simulink library "lib_gyro_fusion"  (R2014a)
settings: Solver=ode45  StartTime=0.0  StopTime=10.0  RelTol=1e-3
undefined symbols (not defined in the file): acc_I, omega_B_noise, omega_bias_I_noise, q_noise, R_gyro
libraries: lib_gyro_fusion x16, aerolibnav x1, simulink x1, vrlib x1
settings Model: Creator=kirill  LastModifiedBy=kirill

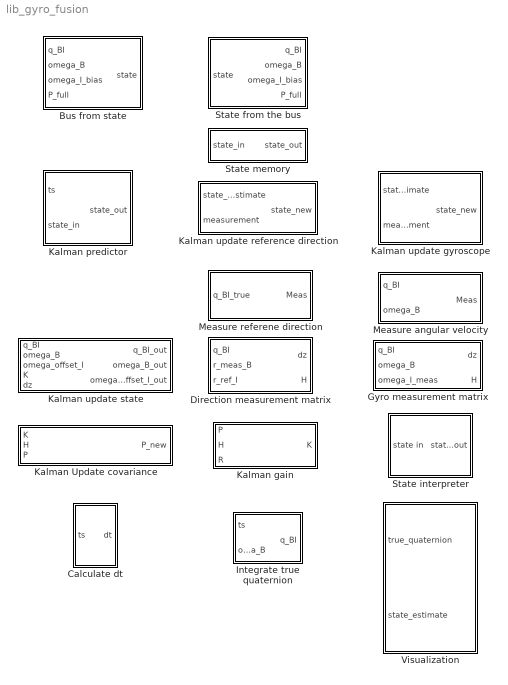
== system lib_gyro_fusion ==
  Bus from state : Subsystem
  Calculate dt : Subsystem
  Direction measurement matrix : Subsystem
  Gyro measurement matrix : Subsystem
  Integrate true quaternion : Subsystem  mask{q_BI_init=[1; 0; 0; 0]}
      mask prompts: q_BI_init "Initial quaternion"
  Kalman Update covariance : MATLAB Function  TreatAsAtomicUnit=on
  Kalman gain : MATLAB Function  TreatAsAtomicUnit=on
  Kalman predictor : Subsystem  mask{q_noise=q_noise, omega_B_noise=omega_B_noise, omega_I_bias_noise=omega_bias_I_noise}
      mask prompts: q_noise "Quaternion dynamics noise [rad/s]"; omega_B_noise "Angular velocity noise [x, y, z], [rad/s^2]"; omega_I_bias_noise "Angular velocity offset noise [rad/s^2]"
  Kalman update gyroscope : Subsystem
  Kalman update reference direction : Subsystem
  Kalman update state : Subsystem
  Measure angular velocity : Subsystem
  Measure referene direction : Subsystem  mask{ref_direction=[1; 0; 0], measurement_noise_power=[1, 1, 1] * 1e-4, measurement_sample_rate=0.1, source_seeds=[340901, 234090, 334090], R_direction=eye(3)}
      mask prompts: ref_direction "Reference direction (inertial frame)"; measurement_noise_power "Measurement noise power"; measurement_sample_rate "Measurement sample rate (seconds)"; source_seeds "Measurement random seeds"; R_direction "Direction measurement covariance covariance"
  State from the bus : Subsystem
  State interpreter : Subsystem
  State memory : Subsystem  mask{q_BI_init=[1; 0; 0; 0], omega_B_init=[0; 0; 0], omega_I_bias_init=[0; 0; 0], P_full_init=eye(9)}
      mask prompts: q_BI_init "Initial quaternion q_BI (4-column vector)"; omega_B_init "Initial body frame angular velocity"; omega_I_bias_init "Initial gyroscope bias (inertial reference frame)"; P_full_init "Initial full state covariance (9x9)"
  Visualization : Subsystem

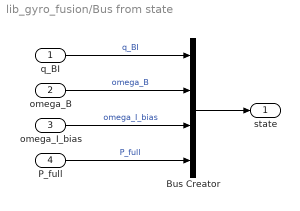
== system lib_gyro_fusion/Bus from state ==
  q_BI : Inport
  omega_B : Inport  Port=2
  omega_I_bias : Inport  Port=3
  P_full : Inport  Port=4
  Bus Creator : BusCreator
  state : Outport
  wires:
  omega_I_bias/1 -> Bus Creator/3  "omega_I_bias"
  P_full/1 -> Bus Creator/4  "P_full"
  q_BI/1 -> Bus Creator/1  "q_BI"
  omega_B/1 -> Bus Creator/2  "omega_B"
  Bus Creator/1 -> state/1

== system lib_gyro_fusion/Calculate dt ==
  ts : Inport
  Calculate dt : Sum  Inputs=+-
  Unit Delay : UnitDelay  SampleTime=-1
  dt : Outport
  wires:
  Unit Delay/1 -> Calculate dt/2
  Calculate dt/1 -> dt/1
  ts/1 -> Calculate dt/1, Unit Delay/1

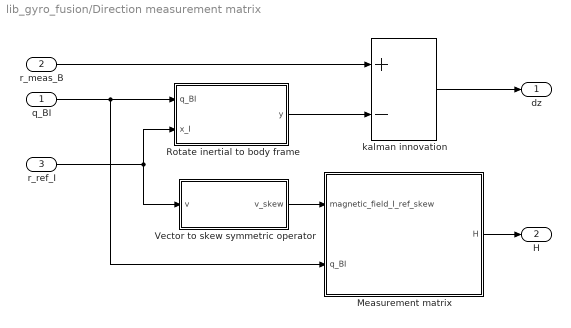
== system lib_gyro_fusion/Direction measurement matrix ==
  q_BI : Inport
  r_meas_B : Inport  Port=2
  r_ref_I : Inport  Port=3
  Measurement matrix : MATLAB Function  TreatAsAtomicUnit=on
  Rotate inertial to body frame : MATLAB Function  TreatAsAtomicUnit=on
  Vector to skew symmetric operator : MATLAB Function  TreatAsAtomicUnit=on
  kalman innovation : Sum  Inputs=+-
  dz : Outport
  H : Outport  Port=2
  wires:
  q_BI/1 -> Measurement matrix/2(q_BI), Rotate inertial to body frame/1(q_BI)
  r_ref_I/1 -> Rotate inertial to body frame/2(x_I), Vector to skew symmetric operator/1(v)
  Rotate inertial to body frame/1(y) -> kalman innovation/2
  r_meas_B/1 -> kalman innovation/1
  kalman innovation/1 -> dz/1
  Vector to skew symmetric operator/1(v_skew) -> Measurement matrix/1(magnetic_field_I_ref_skew)
  Measurement matrix/1(H) -> H/1

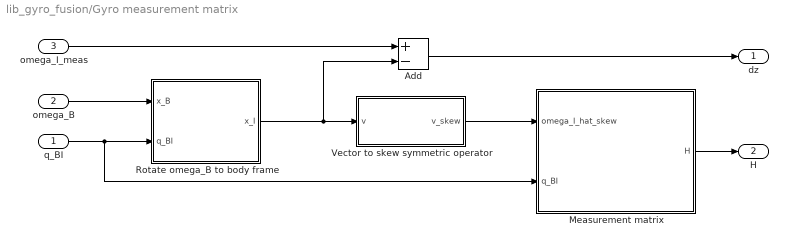
== system lib_gyro_fusion/Gyro measurement matrix ==
  q_BI : Inport
  omega_B : Inport  Port=2
  omega_I_meas : Inport  Port=3
  Add : Sum  Inputs=+-
  Measurement matrix : MATLAB Function  TreatAsAtomicUnit=on
  Rotate omega_B to body frame : MATLAB Function  TreatAsAtomicUnit=on
  Vector to skew symmetric operator : MATLAB Function  TreatAsAtomicUnit=on
  dz : Outport
  H : Outport  Port=2
  wires:
  Add/1 -> dz/1
  omega_I_meas/1 -> Add/1
  q_BI/1 -> Rotate omega_B to body frame/2(q_BI), Measurement matrix/2(q_BI)
  Vector to skew symmetric operator/1(v_skew) -> Measurement matrix/1(omega_I_hat_skew)
  Measurement matrix/1(H) -> H/1
  Rotate omega_B to body frame/1(x_I) -> Add/2, Vector to skew symmetric operator/1(v)
  omega_B/1 -> Rotate omega_B to body frame/1(x_B)

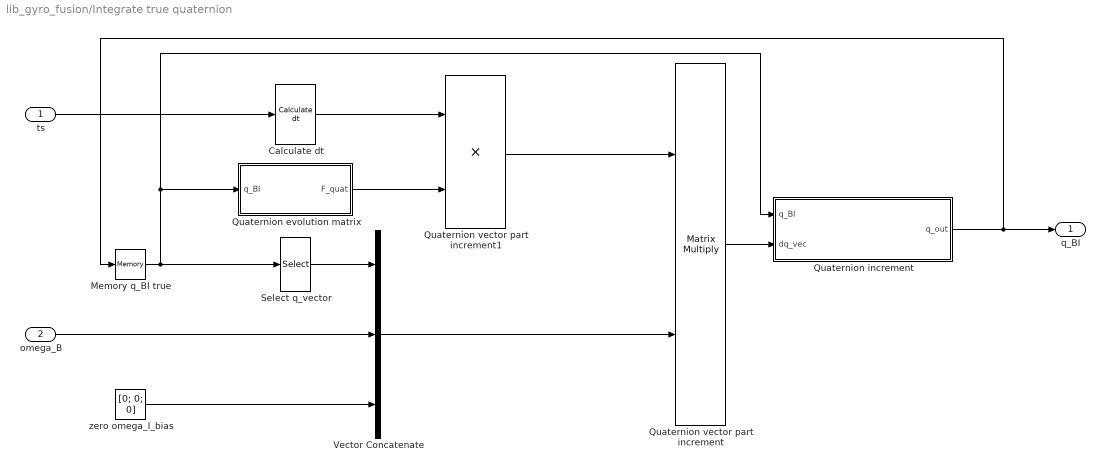
== system lib_gyro_fusion/Integrate true quaternion ==
  ts : Inport
  omega_B : Inport  Port=2
  Calculate dt : lib_gyro_fusion/Calculate dt
  Memory q_BI true : Memory  X0=q_BI_init
  Quaternion evolution matrix : MATLAB Function  TreatAsAtomicUnit=on
  Quaternion increment : MATLAB Function  TreatAsAtomicUnit=on
  Quaternion vector part increment : Product  Multiplication=Matrix(*)
  Quaternion vector part increment1 : Product
  Select q_vector : Selector  InputPortWidth=4  IndexOptions=Starting index (dialog)  Indices=2  OutputSizes=3
  Vector Concatenate : Concatenate  NumInputs=3
  zero omega_I_bias : Constant  Value=[0; 0; 0]
  q_BI : Outport
  wires:
  Quaternion vector part increment/1 -> Quaternion increment/2(dq_vec)
  zero omega_I_bias/1 -> Vector Concatenate/3
  Vector Concatenate/1 -> Quaternion vector part increment/2
  omega_B/1 -> Vector Concatenate/2
  Quaternion evolution matrix/1(F_quat) -> Quaternion vector part increment1/2
  Calculate dt/1 -> Quaternion vector part increment1/1
  Quaternion increment/1(q_out) -> q_BI/1, Memory q_BI true/1
  Memory q_BI true/1 -> Quaternion increment/1(q_BI), Quaternion evolution matrix/1(q_BI), Select q_vector/1
  Quaternion vector part increment1/1 -> Quaternion vector part increment/1
  ts/1 -> Calculate dt/1
  Select q_vector/1 -> Vector Concatenate/1

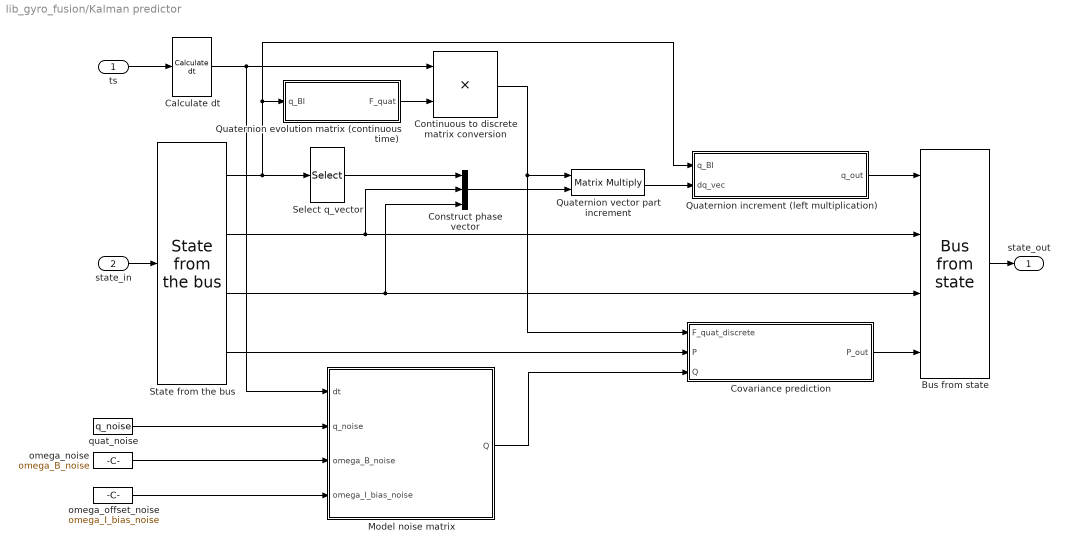
== system lib_gyro_fusion/Kalman predictor ==
  ts : Inport
  state_in : Inport  Port=2
  Bus from state : lib_gyro_fusion/Bus from state
  Calculate dt : lib_gyro_fusion/Calculate dt
  Construct phase vector : Concatenate  NumInputs=3
  Continuous to discrete matrix conversion : Product
  Covariance prediction : MATLAB Function  TreatAsAtomicUnit=on
  Model noise matrix : MATLAB Function  TreatAsAtomicUnit=on
  Quaternion evolution matrix (continuous time) : MATLAB Function  TreatAsAtomicUnit=on
  Quaternion increment (left multiplication) : MATLAB Function  TreatAsAtomicUnit=on
  Quaternion vector part increment : Product  Multiplication=Matrix(*)
  Select q_vector : Selector  InputPortWidth=4  IndexOptions=Starting index (dialog)  Indices=2  OutputSizes=3
  State from the bus : lib_gyro_fusion/State from the bus
  omega_noise : Constant  Value=omega_B_noise
  omega_offset_noise : Constant  Value=omega_I_bias_noise
  quat_noise : Constant  Value=q_noise
  state_out : Outport
  wires:
  omega_offset_noise/1 -> Model noise matrix/4(omega_I_bias_noise)
  omega_noise/1 -> Model noise matrix/3(omega_B_noise)
  Calculate dt/1 -> Continuous to discrete matrix conversion/1, Model noise matrix/1(dt)
  quat_noise/1 -> Model noise matrix/2(q_noise)
  Model noise matrix/1(Q) -> Covariance prediction/3(Q)
  Covariance prediction/1(P_out) -> Bus from state/4
  State from the bus/4 -> Covariance prediction/2(P)
  Construct phase vector/1 -> Quaternion vector part increment/2
  Continuous to discrete matrix conversion/1 -> Quaternion vector part increment/1, Covariance prediction/1(F_quat_discrete)
  Quaternion evolution matrix (continuous time)/1(F_quat) -> Continuous to discrete matrix conversion/2
  Quaternion vector part increment/1 -> Quaternion increment (left multiplication)/2(dq_vec)
  Select q_vector/1 -> Construct phase vector/1
  State from the bus/1 -> Select q_vector/1, Quaternion evolution matrix (continuous time)/1(q_BI), Quaternion increment (left multiplication)/1(q_BI)
  ts/1 -> Calculate dt/1
  Quaternion increment (left multiplication)/1(q_out) -> Bus from state/1
  State from the bus/2 -> Construct phase vector/2, Bus from state/2
  State from the bus/3 -> Bus from state/3, Construct phase vector/3
  Bus from state/1 -> state_out/1
  state_in/1 -> State from the bus/1

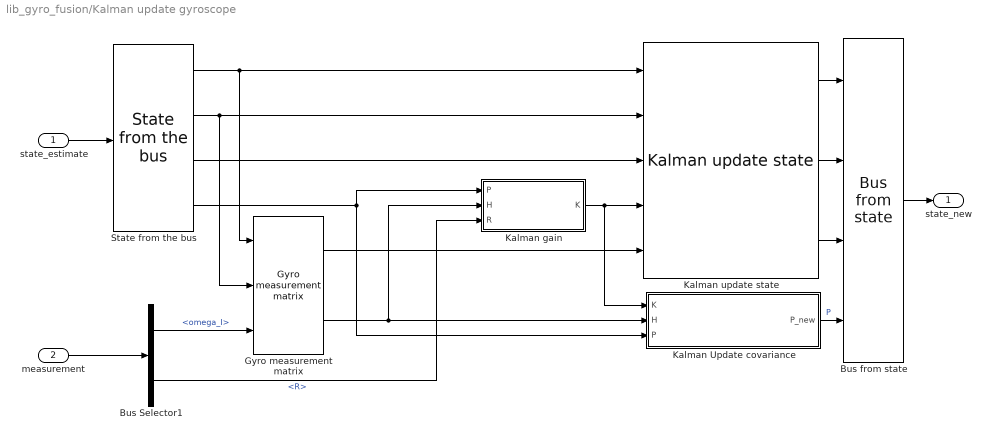
== system lib_gyro_fusion/Kalman update gyroscope ==
  state_estimate : Inport
  measurement : Inport  Port=2
  Bus Selector1 : BusSelector  OutputSignals=omega_I,R
  Bus from state : lib_gyro_fusion/Bus from state
  Gyro measurement matrix : lib_gyro_fusion/Gyro measurement matrix
  Kalman Update covariance : MATLAB Function  TreatAsAtomicUnit=on
  Kalman gain : MATLAB Function  TreatAsAtomicUnit=on
  Kalman update state : lib_gyro_fusion/Kalman update state
  State from the bus : lib_gyro_fusion/State from the bus
  state_new : Outport
  wires:
  Kalman update state/2 -> Bus from state/2
  Bus Selector1/2 -> Kalman gain/3(R)  "<R>"
  Kalman update state/3 -> Bus from state/3
  Kalman update state/1 -> Bus from state/1
  Gyro measurement matrix/1 -> Kalman update state/5
  Kalman gain/1(K) -> Kalman update state/4, Kalman Update covariance/1(K)
  State from the bus/3 -> Kalman update state/3
  State from the bus/2 -> Gyro measurement matrix/2, Kalman update state/2
  Gyro measurement matrix/2 -> Kalman gain/2(H), Kalman Update covariance/2(H)
  Bus Selector1/1 -> Gyro measurement matrix/3  "<omega_I>"
  State from the bus/1 -> Gyro measurement matrix/1, Kalman update state/1
  State from the bus/4 -> Kalman gain/1(P), Kalman Update covariance/3(P)
  state_estimate/1 -> State from the bus/1
  measurement/1 -> Bus Selector1/1
  Kalman Update covariance/1(P_new) -> Bus from state/4  "P"
  Bus from state/1 -> state_new/1

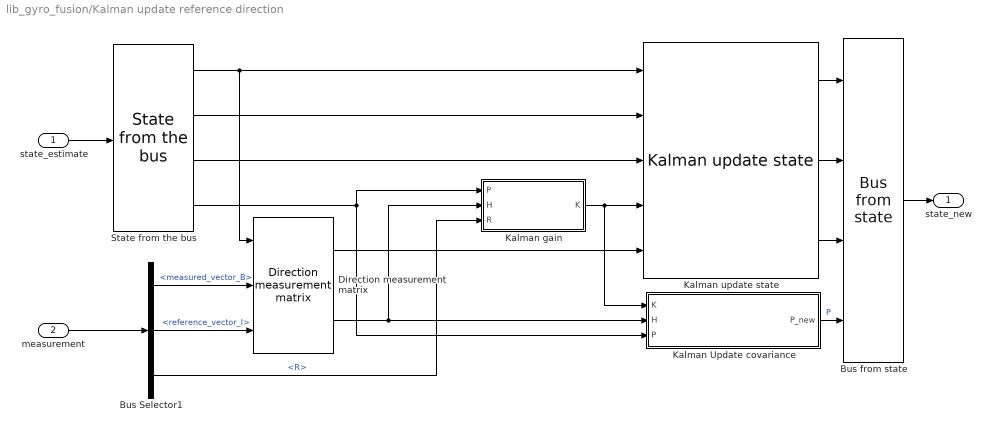
== system lib_gyro_fusion/Kalman update reference direction ==
  state_estimate : Inport
  measurement : Inport  Port=2
  Bus Selector1 : BusSelector  OutputSignals=measured_vector_B,reference_vector_I,R
  Bus from state : lib_gyro_fusion/Bus from state
  Direction measurement matrix : lib_gyro_fusion/Direction measurement matrix
  Kalman Update covariance : MATLAB Function  TreatAsAtomicUnit=on
  Kalman gain : MATLAB Function  TreatAsAtomicUnit=on
  Kalman update state : lib_gyro_fusion/Kalman update state
  State from the bus : lib_gyro_fusion/State from the bus
  state_new : Outport
  wires:
  Bus from state/1 -> state_new/1
  Kalman Update covariance/1(P_new) -> Bus from state/4  "P"
  measurement/1 -> Bus Selector1/1
  state_estimate/1 -> State from the bus/1
  State from the bus/4 -> Kalman Update covariance/3(P), Kalman gain/1(P)
  State from the bus/1 -> Direction measurement matrix/1, Kalman update state/1
  Bus Selector1/1 -> Direction measurement matrix/2  "<measured_vector_B>"
  Bus Selector1/2 -> Direction measurement matrix/3  "<reference_vector_I>"
  Direction measurement matrix/2 -> Kalman Update covariance/2(H), Kalman gain/2(H)
  State from the bus/2 -> Kalman update state/2
  State from the bus/3 -> Kalman update state/3
  Kalman gain/1(K) -> Kalman Update covariance/1(K), Kalman update state/4
  Direction measurement matrix/1 -> Kalman update state/5
  Kalman update state/1 -> Bus from state/1
  Kalman update state/3 -> Bus from state/3
  Bus Selector1/3 -> Kalman gain/3(R)  "<R>"
  Kalman update state/2 -> Bus from state/2

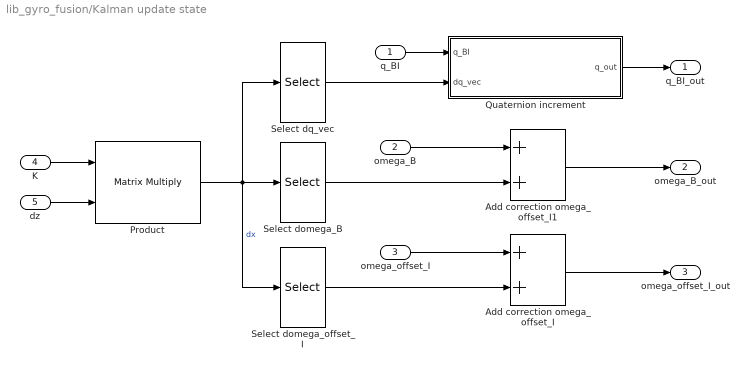
== system lib_gyro_fusion/Kalman update state ==
  q_BI : Inport
  omega_B : Inport  Port=2
  omega_offset_I : Inport  Port=3
  K : Inport  Port=4
  dz : Inport  Port=5
  Add correction omega_offset_I : Sum
  Add correction omega_offset_I1 : Sum
  Product : Product  Multiplication=Matrix(*)
  Quaternion increment : MATLAB Function  TreatAsAtomicUnit=on
  Select domega_B : Selector  InputPortWidth=9  Indices=4:6  OutputSizes=3
  Select domega_offset_I : Selector  InputPortWidth=9  Indices=7:9  OutputSizes=3
  Select dq_vec : Selector  InputPortWidth=9  Indices=1:3  OutputSizes=3
  q_BI_out : Outport
  omega_B_out : Outport  Port=2
  omega_offset_I_out : Outport  Port=3
  wires:
  Quaternion increment/1(q_out) -> q_BI_out/1
  K/1 -> Product/1
  dz/1 -> Product/2
  Product/1 -> Select dq_vec/1, Select domega_B/1, Select domega_offset_I/1  "dx"
  Select dq_vec/1 -> Quaternion increment/2(dq_vec)
  Add correction omega_offset_I1/1 -> omega_B_out/1
  Add correction omega_offset_I/1 -> omega_offset_I_out/1
  Select domega_offset_I/1 -> Add correction omega_offset_I/2
  omega_B/1 -> Add correction omega_offset_I1/1
  q_BI/1 -> Quaternion increment/1(q_BI)
  omega_offset_I/1 -> Add correction omega_offset_I/1
  Select domega_B/1 -> Add correction omega_offset_I1/2

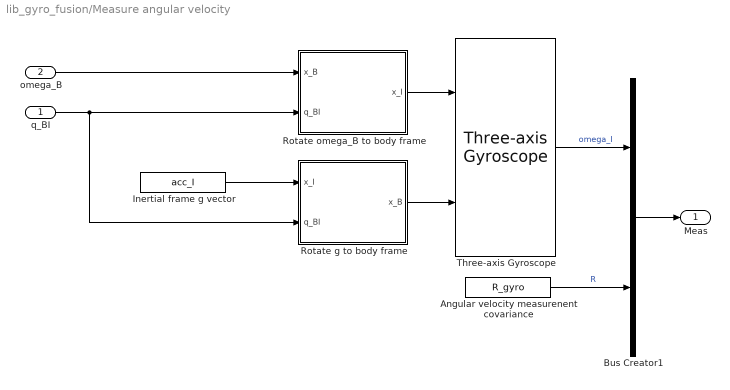
== system lib_gyro_fusion/Measure angular velocity ==
  q_BI : Inport
  omega_B : Inport  Port=2
  Angular velocity measurenent covariance : Constant  Value=R_gyro
  Bus Creator1 : BusCreator  Inputs=2
  Inertial frame g vector : Constant  Value=acc_I
  Rotate g to body frame : MATLAB Function  TreatAsAtomicUnit=on
  Rotate omega_B to body frame : MATLAB Function  TreatAsAtomicUnit=on
  Three-axis Gyroscope : aerolibnav/Three-axis Gyroscope  dtype_g=on  w_g=gyro_natrual_freq  z_g=gyro_damping_factor  g_sf_cc=gyro_scale_factor  g_bias=gyro_mean_bias  g_sen=gyro_g_sensitivity_bias  g_rand=on  g_seeds=gyro_seeds  g_pow=gyro_noise  g_sat="[-inf  -inf  -inf  inf inf inf]"  g_Ts=t_step
  Meas : Outport
  wires:
  Angular velocity measurenent covariance/1 -> Bus Creator1/2  "R"
  Bus Creator1/1 -> Meas/1
  Three-axis Gyroscope/1 -> Bus Creator1/1  "omega_I"
  omega_B/1 -> Rotate omega_B to body frame/1(x_B)
  q_BI/1 -> Rotate g to body frame/2(q_BI), Rotate omega_B to body frame/2(q_BI)
  Rotate omega_B to body frame/1(x_I) -> Three-axis Gyroscope/1
  Inertial frame g vector/1 -> Rotate g to body frame/1(x_I)
  Rotate g to body frame/1(x_B) -> Three-axis Gyroscope/2

== system lib_gyro_fusion/Measure referene direction ==
  q_BI_true : Inport
  Bus Creator1 : BusCreator  Inputs=3
  Magnetic field measurement covariance : Constant  Value=R_direction
  Magnetometer : Subsystem
  Reference field : Constant  Value=ref_direction
  Meas : Outport
  wires:
  Magnetic field measurement covariance/1 -> Bus Creator1/3  "R"
  Magnetometer/1(Meas) -> Bus Creator1/1  "measured_vector_B"
  Reference field/1 -> Bus Creator1/2, Magnetometer/2(ref_I)  "reference_vector_I"
  Bus Creator1/1 -> Meas/1
  q_BI_true/1 -> Magnetometer/1(q_BI)

== system lib_gyro_fusion/State from the bus ==
  state : Inport
  Bus Selector : BusSelector  OutputSignals=q_BI,omega_B,omega_I_bias,P_full
  q_BI : Outport
  omega_B : Outport  Port=2
  omega_I_bias : Outport  Port=3
  P_full : Outport  Port=4
  wires:
  Bus Selector/1 -> q_BI/1  "<q_BI>"
  Bus Selector/4 -> P_full/1  "<P_full>"
  Bus Selector/3 -> omega_I_bias/1  "<omega_I_bias>"
  state/1 -> Bus Selector/1
  Bus Selector/2 -> omega_B/1  "<omega_B>"

== system lib_gyro_fusion/State interpreter ==
  state in : Inport
  Bias removal : Sum  Inputs=+-
  Bus from state : lib_gyro_fusion/Bus from state
  I2B1 : MATLAB Function  TreatAsAtomicUnit=on
  State from the bus : lib_gyro_fusion/State from the bus
  state_out : Outport
  wires:
  State from the bus/4 -> Bus from state/4
  I2B1/1(omega_B) -> Bias removal/2
  State from the bus/2 -> Bias removal/1
  state in/1 -> State from the bus/1
  Bus from state/1 -> state_out/1
  Bias removal/1 -> Bus from state/2
  State from the bus/1 -> I2B1/1(q_BI), Bus from state/1
  State from the bus/3 -> I2B1/2(omega_I), Bus from state/3

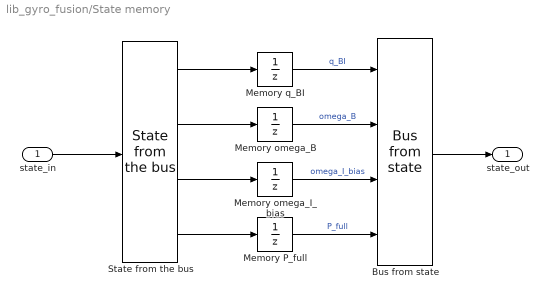
== system lib_gyro_fusion/State memory ==
  state_in : Inport
  Bus from state : lib_gyro_fusion/Bus from state
  Memory P_full : UnitDelay  InitialCondition=P_full_init  SampleTime=-1
  Memory omega_B : UnitDelay  InitialCondition=omega_B_init  SampleTime=-1
  Memory omega_I_bias : UnitDelay  InitialCondition=omega_I_bias_init  SampleTime=-1
  Memory q_BI : UnitDelay  InitialCondition=q_BI_init  SampleTime=-1
  State from the bus : lib_gyro_fusion/State from the bus
  state_out : Outport
  wires:
  Memory q_BI/1 -> Bus from state/1  "q_BI"
  State from the bus/2 -> Memory omega_B/1
  State from the bus/4 -> Memory P_full/1
  Bus from state/1 -> state_out/1
  State from the bus/1 -> Memory q_BI/1
  state_in/1 -> State from the bus/1
  Memory omega_I_bias/1 -> Bus from state/3  "omega_I_bias"
  Memory omega_B/1 -> Bus from state/2  "omega_B"
  State from the bus/3 -> Memory omega_I_bias/1
  Memory P_full/1 -> Bus from state/4  "P_full"

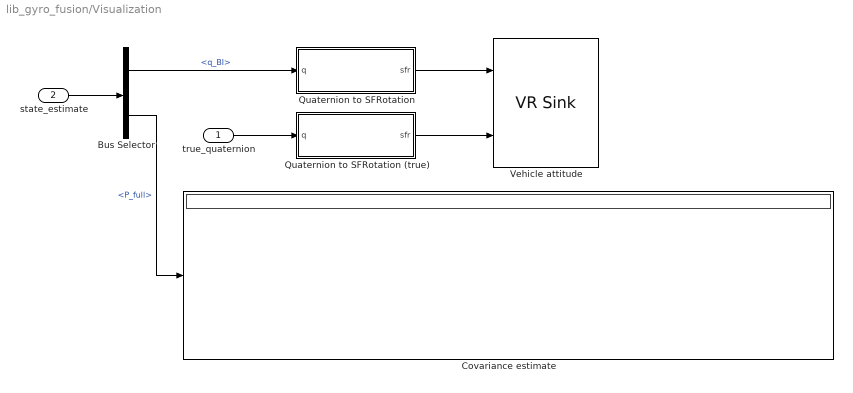
== system lib_gyro_fusion/Visualization ==
  true_quaternion : Inport
  state_estimate : Inport  Port=2
  Bus Selector : BusSelector  OutputSignals=q_BI,P_full
  Covariance estimate : Display
  Quaternion to SFRotation : MATLAB Function  TreatAsAtomicUnit=on
  Quaternion to SFRotation (true) : MATLAB Function  TreatAsAtomicUnit=on
  Vehicle attitude : vrlib/VR Sink  InstantiateOnLoad=on  SampleTime=0.1  ViewEnable=on  RemoteChange=off  RemoteView=off  FieldsWritten=Estimated_car.rotation.4.1.1.double#True_car.rotation.4.1.1.double  WorldFileName=ins.wrl  AutoView=off  VideoDimensions=[]  AllowVariableSize=off
  wires:
  Bus Selector/2 -> Covariance estimate/1  "<P_full>"
  state_estimate/1 -> Bus Selector/1
  Bus Selector/1 -> Quaternion to SFRotation/1(q)  "<q_BI>"
  Quaternion to SFRotation (true)/1(sfr) -> Vehicle attitude/2
  Quaternion to SFRotation/1(sfr) -> Vehicle attitude/1
  true_quaternion/1 -> Quaternion to SFRotation (true)/1(q)

== system lib_gyro_fusion/Measure referene direction/Magnetometer ==
  q_BI : Inport
  ref_I : Inport  Port=2
  Add : Sum
  Noise source : simulink/Sources/Band-Limited White Noise  Cov=measurement_noise_power  Ts=measurement_sample_rate  seed=source_seeds
  Rotate inertial to body frame : MATLAB Function  TreatAsAtomicUnit=on
  Meas : Outport
  wires:
  q_BI/1 -> Rotate inertial to body frame/2(q_BI)
  Add/1 -> Meas/1
  Noise source/1 -> Add/2
  Rotate inertial to body frame/1(x_B) -> Add/1
  ref_I/1 -> Rotate inertial to body frame/1(x_I)

== matlab function lib_gyro_fusion/Kalman predictor/Covariance prediction ==
  data: F_quat_discrete input; P input; P_out output; Q input
function P_out = F_cont(F_quat_discrete, P, Q)
%#codegen
F = eye(9);
F(1:3, :) = F(1:3, :) + F_quat_discrete;
P_out = F * P * F' + Q;

== matlab function lib_gyro_fusion/Kalman Update covariance ==
  data: K input; P_new output; H input; P input
function P_new = kalman_update_covariance(K, H, P)
%#codegen
P_new = (eye(9) - K * H) * P;

== matlab function lib_gyro_fusion/Kalman predictor/Model noise matrix ==
  data: dt input; q_noise input; omega_B_noise input; omega_I_bias_noise input; Q output
function Q = Q_discrete(dt, q_noise, omega_B_noise, omega_I_bias_noise)
%#codegen
Q = diag([ ...
    ones(1, 3) * q_noise^2 * dt^2 / 2, ... Quternion evolution noise
    (omega_B_noise.^2)' * dt, ... Angular velocity evolution noise covariance
    ones(1, 3) * omega_I_bias_noise^2 * dt ... Gyro drift noise covariance
    ]);

== matlab function lib_gyro_fusion/Integrate true quaternion/Quaternion evolution matrix ==
  data: F_quat output; q_BI input
function F_quat = F_discrete(q_BI)
% Generate kalman evolution matrix as F = F_cont * dt + E, where F_cont
% represents linearized dynamics matrix \dot{x} = Fx
%#codegen
F_quat = quaternionLinearizedDynamics(q_BI);

== matlab function lib_gyro_fusion/Integrate true quaternion/Quaternion increment ==
  data: q_BI input; dq_vec input; q_out output
function q_out = quaternion_increment(q_BI, dq_vec)
%#codegen

dq = [sqrt(1 - norm(dq_vec)^2); dq_vec];
q_out = quaternionMultiply(dq, q_BI);
% Every time the quaternion is updated it should be re-normalized
q_out = q_out / norm(q_out);

== matlab function lib_gyro_fusion/Kalman update state/Quaternion increment ==
  data: q_BI input; dq_vec input; q_out output
function q_out = quaternion_increment(q_BI, dq_vec)
%#codegen
dq = [1; dq_vec];
dq = dq / norm(dq);
q_out = quaternionMultiply(dq, q_BI);
% Every time the quaternion is updated it should be re-normalized
q_out = q_out / norm(q_out);

== matlab function lib_gyro_fusion/Direction measurement matrix/Rotate inertial to body frame ==
  data: q_BI input; x_I input; y output
function y = transofrmI2B(q_BI, x_I)
% Rotate vector from ECI to fixed reference frame if q represents body
% orientation in ECI reference frame
%#codegen
y = rotateI2B(x_I, q_BI);

== matlab function lib_gyro_fusion/Direction measurement matrix/Vector to skew symmetric operator ==
  data: v input; v_skew output
function v_skew = vec2skew_sym(v)
%#codegen
v_skew = vector2antiSkewSymOperator(v);

== matlab function lib_gyro_fusion/Kalman update reference direction/Kalman Update covariance ==
  data: K input; P_new output; H input; P input
function P_new = kalman_update_covariance(K, H, P)
%#codegen
P_new = (eye(9) - K * H) * P;

== matlab function lib_gyro_fusion/Kalman update reference direction/Kalman gain ==
  data: P input; H input; R input; K output
function K  = kalman_gain(P, H, R)
%#codegen
% Calculate total kalman covariance
S = H * P * H' + R;
S_inv = inv(S);
% Calculate Kalman gain matrix
K = P * H' * S_inv;

== matlab function lib_gyro_fusion/Kalman predictor/Quaternion evolution matrix (continuous time) ==
  data: F_quat output; q_BI input
function F_quat = F_cont(q_BI)
% Generate kalman evolution matrix as F = F_cont * dt + E, where F_cont
% represents linearized dynamics matrix \dot{x} = Fx
%#codegen
F_quat = quaternionLinearizedDynamics(q_BI);

== matlab function lib_gyro_fusion/Kalman predictor/Quaternion increment (left multiplication) ==
  data: q_BI input; dq_vec input; q_out output
function q_out = quaternion_increment(q_BI, dq_vec)
%#codegen

dq = [1; dq_vec];
dq = dq / norm(dq);
q_out = quaternionMultiply(dq, q_BI);
% Every time the quaternion is updated it should be re-normalized
q_out = q_out / norm(q_out);

== matlab function lib_gyro_fusion/Gyro measurement matrix/Measurement matrix ==
  data: omega_I_hat_skew input; H output; q_BI input
function H = kalman_update(omega_I_hat_skew, q_BI)
%#codegen
H = gyroMeasurementMatrix(q_BI, omega_I_hat_skew);

== matlab function lib_gyro_fusion/Gyro measurement matrix/Rotate omega_B to body frame ==
  data: x_I output; x_B input; q_BI input
function x_I = transformB2I(x_B, q_BI)
% Rotate vector from ECI to fixed reference frame if q represents body
% orientation in ECI reference frame

%#codegen
x_I = rotateB2I(x_B, q_BI);

== matlab function lib_gyro_fusion/Gyro measurement matrix/Vector to skew symmetric operator ==
  data: v input; v_skew output
function v_skew = vec2skew_sym(v)
%#codegen
v_skew = vector2antiSkewSymOperator(v);

== matlab function lib_gyro_fusion/Kalman update gyroscope/Kalman Update covariance ==
  data: K input; P_new output; H input; P input
function P_new = kalman_update_covariance(K, H, P)
%#codegen
P_new = (eye(9) - K * H) * P;

== matlab function lib_gyro_fusion/Direction measurement matrix/Measurement matrix ==
  data: magnetic_field_I_ref_skew input; H output; q_BI input
function H = kalman_update(magnetic_field_I_ref_skew, q_BI)
%#codegen
H = directionMeasurementMatrix(magnetic_field_I_ref_skew, q_BI);

== matlab function lib_gyro_fusion/Kalman gain ==
  data: P input; H input; R input; K output
function K  = kalman_gain(P, H, R)
%#codegen
% Calculate total kalman covariance
S = H * P * H' + R;
S_inv = inv(S);
% Calculate Kalman gain matrix
K = P * H' * S_inv;

== matlab function lib_gyro_fusion/Kalman update gyroscope/Kalman gain ==
  data: P input; H input; R input; K output
function K  = kalman_gain(P, H, R)
%#codegen
% Calculate total kalman covariance
S = H * P * H' + R;
S_inv = inv(S);
% Calculate Kalman gain matrix
K = P * H' * S_inv;

== matlab function lib_gyro_fusion/Measure angular velocity/Rotate g to body frame ==
  data: x_I input; x_B output; q_BI input
function x_B = transformI2B(x_I, q_BI)
% Rotate vector from ECI to fixed reference frame if q represents body
% orientation in ECI reference frame

%#codegen
x_B = rotateI2B(x_I, q_BI);

== matlab function lib_gyro_fusion/Measure angular velocity/Rotate omega_B to body frame ==
  data: x_I output; x_B input; q_BI input
function x_I = transformB2I(x_B, q_BI)
% Rotate vector from ECI to fixed reference frame if q represents body
% orientation in ECI reference frame

%#codegen
x_I = rotateB2I(x_B, q_BI);

== matlab function lib_gyro_fusion/State interpreter/I2B1 ==
  data: q_BI input; omega_B output; omega_I input
function omega_B = I2B(q_BI, omega_I)
%#codegen
omega_B = rotateI2B(omega_I, q_BI);

== matlab function lib_gyro_fusion/Visualization/Quaternion to SFRotation ==
  data: q input; sfr output
function sfr = quaternion2rotation(q)
%#codegen

sfr = zeros(size(q));
sfr(1:3) = q(2:4);
sfr(4) = 2 * acos(q(1));

== matlab function lib_gyro_fusion/Visualization/Quaternion to SFRotation (true) ==
  data: q input; sfr output
function sfr = quaternion2rotation(q)
%#codegen

sfr = zeros(size(q));
sfr(1:3) = q(2:4);
sfr(4) = 2 * acos(q(1));

== matlab function lib_gyro_fusion/Measure referene direction/Magnetometer/Rotate inertial to body frame ==
  data: x_I input; x_B output; q_BI input
function x_B = transformI2B(x_I, q_BI)
% Rotate vector from ECI to fixed reference frame if q represents body
% orientation in ECI reference frame

%#codegen
x_B = rotateI2B(x_I, q_BI);
